simulink model "DR_Telemedicine_Pipeline"  (R2026a)
settings: Solver=VariableStepAuto
settings Model: Creator=acer  LastModifiedBy=acer

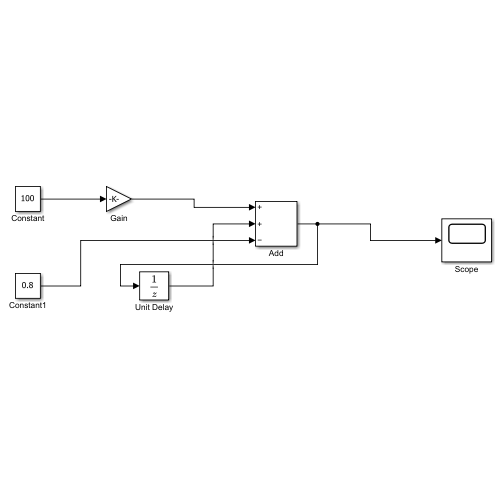
[thumbnail: Simulink's stored preview of the top-level diagram]
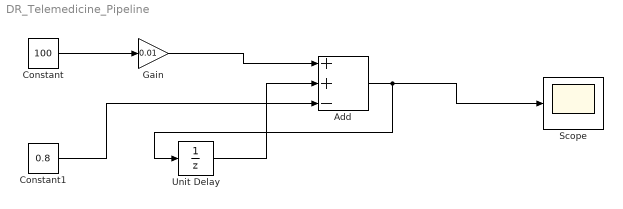
== system DR_Telemedicine_Pipeline ==
  Add : Sum  Inputs=++-
  Constant : Constant  Value=100
  Constant1 : Constant  Value=0.8
  Gain : Gain  Gain=0.01
  Scope : Scope
      settings: ActiveDisplayYMinimum=1.3344360232569716  ActiveDisplayYMaximum=9.6920648110520666
  Unit Delay : UnitDelay  InitialCondition=5  SampleTime=-1
  wires:
  Add/1 -> Unit Delay/1, Scope/1
  Unit Delay/1 -> Add/2
  Constant/1 -> Gain/1
  Gain/1 -> Add/1
  Constant1/1 -> Add/3
